simulink model "env_extQ16"  (R2022b)
settings: Solver=VariableStepAuto  StartTime=0.0  StopTime=30  RelTol=1e-3
values from neighbouring files (symbols this model uses):
  B = 8    [variables.m]    (also in variables16.m)
  cordic_delay = 20    [variables.m]    (also in variables16.m)
  e_val = 1/l2    [variables.m]    (also in variables16.m)
  exp_fract_len_homo = 26    [variables.m]    (also in variables16.m = 10)
  exp_word_len_homo = 32    [variables.m]    (also in variables16.m = 16)
  explarge_delay = 3    [variables.m]    (also in variables16.m)
  fft_len_hilb = 2048    [variables.m]    (also in variables16.m)
  fft_length = 4096    [variables.m]    (also in variables16.m)
  frac_bit_l2 = 30    [variables.m]    (also in variables16.m = 14)
  frac_bit_l3 = 29    [variables.m]    (also in variables16.m = 13)
  frac_bit_l4 = 28    [variables.m]    (also in variables16.m = 12)
  grp_delay_hilb = 11    [variables.m]    (also in variables16.m)
  grp_delay_homo = 13    [variables.m]    (also in variables16.m)
  grp_delay_psd = 19    [variables.m]    (also in variables16.m)
  grp_delay_swt = 12    [variables.m]    (also in variables16.m)
  l2 = log(2)    [variables.m]    (also in variables16.m)
  l2e = 1/log2(exp(1))    [variables.m]    (also in variables16.m)
  log2_table = log2((2^(B-1) : 2^(B)) / 2^(B - 1))    [variables.m]    (also in variables16.m)
  log_fract_len_homo = 31    [variables.m]    (also in variables16.m = 15)
  log_latency = 21    [variables.m]    (also in variables16.m)
  log_word_len = 48    [variables.m]    (also in variables16.m = 24)
  log_word_len_homo = 32    [variables.m]    (also in variables16.m = 16)
  NLZLUT = B-ceil(log2((1:2^B)))    [variables.m]    (also in variables16.m)
  scale = 1.0 / (fs * sum(window_val.*window_val))    [variables.m]    (also in variables16.m)
  win_dim = 64    [variables.m]    (also in variables16.m)
  window_dim = 100    [variables.m]    (also in variables16.m)
undefined symbols (not defined in the file or in its folder): C, c, fl_high_index, fl_low_index, HiD, hilbert_fifo_full, LoD, psd_fifo_full, SFVC784, swt_fifo_full, XCK26, xlfda_numerator
libraries: hdlBasic x626, hdlDSPIP x12, hdlUtilities x2, dspsnks4 x1, dspvision x1, vmcUtilities x1
(part 4 of 7)

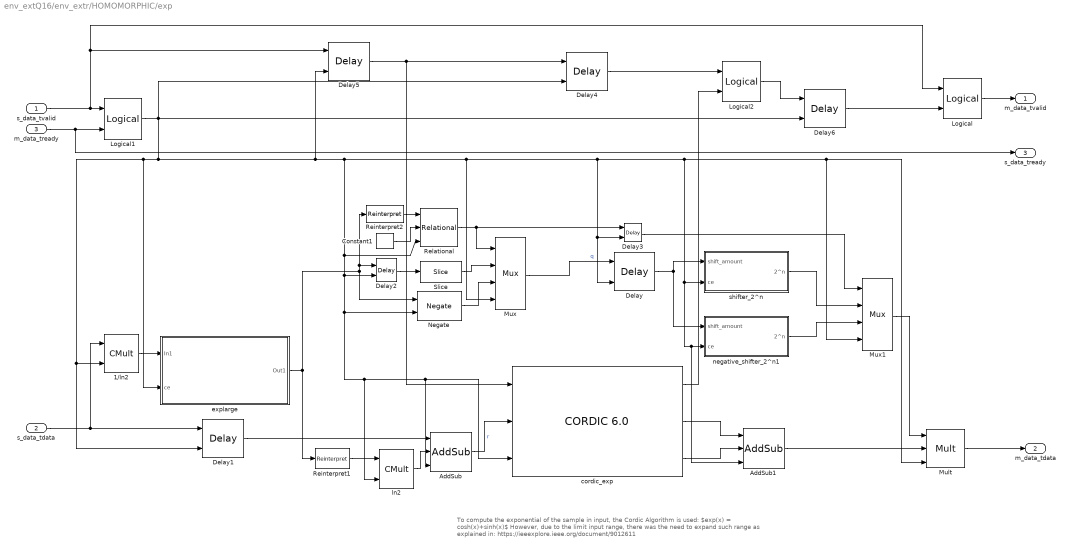
== system env_extQ16/env_extr/HOMOMORPHIC/exp ==
  note: To compute the exponential of the sample in input, the Cordic Algorithm is used: $exp(x) = cosh(x)+sinh(x)$
      |
      | However, due to the limit input range, there was the need to expand such range as explained in:
      | https://ieeexplore.ieee.org/document/9012611
  s_data_tvalid : Inport
  s_data_tdata : Inport  Port=2
  m_data_tready : Inport  Port=3
  1/ln2 : hdlBasic/CMult  const=e_val  gui_display_data_type=Fixed-point  const_n_bits=32  const_bin_pt=30  float_type=Single  exp_bits=8  fraction_bits=24  en=on  latency=1  precision=User Defined  arith_type="Signed  (2's comp)"  n_bits=exp_word_len_homo  bin_pt=exp_fract_len_homo  quantization=Truncate  overflow=Saturate  use_behavioral_HDL=off  mem_type=Distributed RAM  pipeline=off  XmcBlockStatus=1  maskContainerNames=tabcontainer1  block_type=cmult  block_config=sysgen:CMult_config
      settings: infoedit=[]
  AddSub : hdlBasic/AddSub  mode=Subtraction  use_carryin=off  use_carryout=off  en=on  latency=1  precision=User Defined  arith_type="Signed  (2's comp)"  n_bits=cordic_input_width  bin_pt=cordic_bin_point  quantization="Round  (unbiased: +/- Inf)"  overflow=Wrap  use_behavioral_HDL=off  hw_selection=Fabric  pipelined=off  XmcBlockStatus=1  maskContainerNames=tabcontainer1  block_type=addsub  block_config=sysgen:Addsub_config
  AddSub1 : hdlBasic/AddSub  mode=Addition  use_carryin=off  use_carryout=off  en=on  latency=1  precision=Full  arith_type=Unsigned  n_bits=16  bin_pt=14  quantization=Truncate  overflow=Wrap  use_behavioral_HDL=off  hw_selection=Fabric  pipelined=off  XmcBlockStatus=1  maskContainerNames=tabcontainer1  block_type=addsub  block_config=sysgen:Addsub_config
  Constant1 : hdlBasic/Constant  const=0  gui_display_data_type=Fixed-point  arith_type=Signed (2's comp)  n_bits=5  bin_pt=0  preci_type=Single  exp_width=8  frac_width=24  explicit_period=off  period=1  XmcBlockStatus=1  maskContainerNames=tabcontainer1  block_type=constant  block_config=sysgen:Constant_config
  Delay : hdlBasic/Delay  rst=off  en=on  latency=cordic_delay-2  reg_retiming=off  XmcBlockStatus=1  maskContainerNames=group1  block_type=delay  block_config=sysgen:Delay_config
  Delay1 : hdlBasic/Delay  rst=off  en=on  latency=explarge_delay+1+1  reg_retiming=off  XmcBlockStatus=1  maskContainerNames=group1  block_type=delay  block_config=sysgen:Delay_config
  Delay2 : hdlBasic/Delay  rst=off  en=on  latency=1  reg_retiming=off  XmcBlockStatus=1  maskContainerNames=group1  block_type=delay  block_config=sysgen:Delay_config
  Delay3 : hdlBasic/Delay  rst=off  en=on  latency=cordic_delay+1  reg_retiming=off  XmcBlockStatus=1  maskContainerNames=group1  block_type=delay  block_config=sysgen:Delay_config
  Delay4 : hdlBasic/Delay  rst=off  en=on  latency=cordic_delay  reg_retiming=off  XmcBlockStatus=1  maskContainerNames=group1  block_type=delay  block_config=sysgen:Delay_config
  Delay5 : hdlBasic/Delay  rst=off  en=on  latency=6  reg_retiming=off  XmcBlockStatus=1  maskContainerNames=group1  block_type=delay  block_config=sysgen:Delay_config
  Delay6 : hdlBasic/Delay  rst=off  en=on  latency=4  reg_retiming=off  XmcBlockStatus=1  maskContainerNames=group1  block_type=delay  block_config=sysgen:Delay_config
  Logical : hdlBasic/Logical  logical_function=AND  inputs=2  en=off  latency=0  precision=Full  arith_type=Unsigned  n_bits=16  bin_pt=0  align_bp=on  overflow=[]  quantization=[]  XmcBlockStatus=1  maskContainerNames=tabcontainer1  block_type=logical  block_config=sysgen:Logical_config
  Logical1 : hdlBasic/Logical  logical_function=AND  inputs=2  en=off  latency=0  precision=Full  arith_type=Unsigned  n_bits=16  bin_pt=0  align_bp=on  overflow=[]  quantization=[]  XmcBlockStatus=1  maskContainerNames=tabcontainer1  block_type=logical  block_config=sysgen:Logical_config
  Logical2 : hdlBasic/Logical  logical_function=AND  inputs=2  en=off  latency=0  precision=Full  arith_type=Unsigned  n_bits=16  bin_pt=0  align_bp=on  overflow=[]  quantization=[]  XmcBlockStatus=1  maskContainerNames=tabcontainer1  block_type=logical  block_config=sysgen:Logical_config
  Mult : hdlBasic/Mult  precision=User Defined  arith_type="Signed  (2's comp)"  n_bits=32  bin_pt=31  quantization="Round  (unbiased: +/- Inf)"  overflow=Saturate  en=on  latency=3  use_behavioral_HDL=off  opt=Speed  use_embedded=on  optimum_pipeline=off  pipeline=on  use_rpm=on  placement_style=Triangular  XmcBlockStatus=1  maskContainerNames=group1  block_type=mult  block_config=sysgen:Mult_config  block_width=598  block_height=876
  Mux : hdlBasic/Mux  inputs=2  en=on  latency=1  precision=Full  arith_type=Unsigned  n_bits=16  bin_pt=14  quantization=Truncate  overflow=Wrap  XmcBlockStatus=1  maskContainerNames=tabcontainer1  block_type=mux  block_config=sysgen:Mux_config
  Mux1 : hdlBasic/Mux  inputs=2  en=on  latency=1  precision=Full  arith_type=Unsigned  n_bits=16  bin_pt=14  quantization=Truncate  overflow=Wrap  XmcBlockStatus=1  maskContainerNames=tabcontainer1  block_type=mux  block_config=sysgen:Mux_config
  Negate : hdlBasic/Negate  precision=User Defined  arith_type=Unsigned  n_bits=5  bin_pt=0  quantization=Truncate  overflow=Wrap  en=on  latency=1  XmcBlockStatus=1  maskContainerNames=tabcontainer1  block_type=negate  block_config=sysgen:Negate_config
  Reinterpret1 : hdlBasic/Reinterpret  force_arith_type=on  arith_type="Signed  (2's comp)"  force_bin_pt=on  bin_pt=0  XmcBlockStatus=1  maskContainerNames=group1  block_type=reinterpret  block_config=sysgen:Reinterpret_config
  Reinterpret2 : hdlBasic/Reinterpret  force_arith_type=on  arith_type="Signed  (2's comp)"  force_bin_pt=on  bin_pt=0  XmcBlockStatus=1  maskContainerNames=group1  block_type=reinterpret  block_config=sysgen:Reinterpret_config
  Relational : hdlBasic/Relational  mode=a<=b  op_type=Bool  en=on  latency=1  XmcBlockStatus=1  maskContainerNames=tabcontainer1  block_type=relational  block_config=sysgen:Relational_config
  Slice : hdlBasic/Slice  nbits=5  boolean_output=off  mode=Upper Bit Location + Width  bit1=-1  base1=MSB of Input  bit0=0  base0=LSB of Input  XmcBlockStatus=1  maskContainerNames=group1  block_type=slice  block_config=sysgen:Slice_config
  cordic_exp : hdlDSPIP/CORDIC 6.0   functional_selection=Sinh_and_Cosh  architectural_configuration=Parallel  pipelining_mode=Maximum  data_format=SignedFraction  phase_format=Radians  input_width=cordic_input_width  output_width=cordic_output_width  round_mode=Nearest_Even  iterations=cordic_iterations  precision=0  compensation_scaling=No_Scale_Compensation  coarse_rotation=off  aclken=on  aresetn=off  out_tready=off  cartesian_has_tuser=off  cartesian_has_tlast=off  cartesian_tuser_width=1  phase_has_tuser=off  phase_has_tlast=off  phase_tuser_width=1  out_tlast_behv=Null  flow_control=NonBlocking  optimize_goal=Resources  trim_axipin_name=off  simulation_type=hybrid_sim  simulation_model=sysgen:cordic_v6_0  data_path_portlist={'s_axis_cartesian_tdata_imag', 's_axis_cartesian_tdata_real', 's_axis_phase_tdata_phase', 'm_axis_dout_tdata_imag', 'm_axis_dout_tdata_real', 'm_axis_dout_tdata_phase','m_axis_dout_tdata'}  ip_name=CORDIC  ip_version=6.0  dsptool_ready=true  ipcore_usecache=true  ipcore_useipmodelcache=true  wrapper_available=true  port_translation_map={ 'aclken' => 'en', 'aresetn' => 'rst' }  XmcBlockStatus=1  maskContainerNames=group15  block_type=cordic_v6_0  block_config=sysgen:rodinimport_config  block_width=800
  explarge : Subsystem
  ln2 : hdlBasic/CMult  const=l2  gui_display_data_type=Fixed-point  const_n_bits=32  const_bin_pt=31  float_type=Single  exp_bits=8  fraction_bits=24  en=on  latency=1  precision=Full  arith_type="Signed  (2's comp)"  n_bits=33  bin_pt=30  quantization="Round  (unbiased: +/- Inf)"  overflow=Wrap  use_behavioral_HDL=off  mem_type=Distributed RAM  pipeline=off  XmcBlockStatus=1  maskContainerNames=tabcontainer1  block_type=cmult  block_config=sysgen:CMult_config
      settings: infoedit=[]
  negative_shifter_2^n1 : Subsystem
  shifter_2^n : Subsystem
  m_data_tvalid : Outport
  m_data_tdata : Outport  Port=2
  s_data_tready : Outport  Port=3
  wires:
  Slice/1 -> Mux/2
  Reinterpret1/1 -> ln2/1
  s_data_tdata/1 -> 1/ln2/1, Delay1/1
  Delay/1 -> negative_shifter_2^n1/1(shift_amount), shifter_2^n/1(shift_amount)
  Delay2/1 -> Slice/1
  cordic_exp/3 -> AddSub1/2
  Constant1/1 -> Relational/2
  AddSub/1 -> cordic_exp/2  "r"
  explarge/1(Out1) -> Reinterpret1/1, Delay2/1, Reinterpret2/1, Negate/1
  Delay3/1 -> Mux1/1
  Mux1/1 -> Mult/1
  Relational/1 -> Mux/1, Delay3/1
  cordic_exp/2 -> AddSub1/1
  Negate/1 -> Mux/3
  negative_shifter_2^n1/1(2^n) -> Mux1/3
  shifter_2^n/1(2^n) -> Mux1/2
  1/ln2/1 -> explarge/1(In1)
  Mux/1 -> Delay/1  "q"
  Reinterpret2/1 -> Relational/1
  Mult/1 -> m_data_tdata/1
  AddSub1/1 -> Mult/2
  cordic_exp/1 -> Logical2/2
  m_data_tready/1 -> s_data_tready/1, Logical1/2
  s_data_tvalid/1 -> Logical/1, Delay5/1, Logical1/1
  Logical/1 -> m_data_tvalid/1
  Logical1/1 -> Delay4/2, Delay6/2, Delay1/2, 1/ln2/2, explarge/2(ce), Mux/4, Delay/2, Delay3/2, Mux1/4, Mult/3, shifter_2^n/2(ce), negative_shifter_2^n1/2(ce), AddSub1/3, ln2/2, cordic_exp/3, AddSub/3, Negate/2, Delay2/2, Relational/3, Delay5/2
  Delay4/1 -> Logical2/1
  Logical2/1 -> Delay6/1
  Delay6/1 -> Logical/2
  Delay1/1 -> AddSub/1
  ln2/1 -> AddSub/2
  Delay5/1 -> Delay4/1, cordic_exp/1

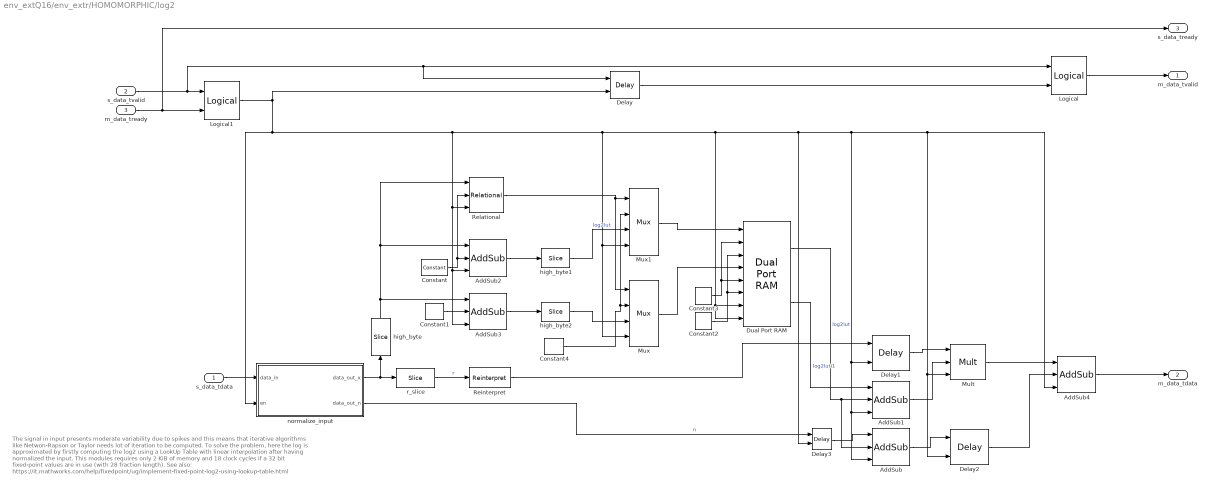
== system env_extQ16/env_extr/HOMOMORPHIC/log2 ==
  note: The signal in input presents moderate variability due to spikes and this means that iterative algorithms like Netwon-Rapson or Taylor needs lot of iteration to be computed.
      |
      | To solve the problem, here the log is approximated by firstly computing the log2 using a LookUp Table with linear interpolation after having normalized the input.
      | This modules requires only 2 KiB of memory and 18 clock cycles if a 32 bit fixed-point values are in use (with 28 fraction length).
      |
      | See also: https://it.mathworks.com/help/fixedpoint/ug/implement-fixed-point-log2-using-lookup-table.html
  s_data_tdata : Inport
  s_data_tvalid : Inport  Port=2
  m_data_tready : Inport  Port=3
  AddSub : hdlBasic/AddSub  mode=Addition  use_carryin=off  use_carryout=off  en=on  latency=1  precision=User Defined  arith_type="Signed  (2's comp)"  n_bits=32  bin_pt=25  quantization="Round  (unbiased: +/- Inf)"  overflow=Wrap  use_behavioral_HDL=off  hw_selection=Fabric  pipelined=off  XmcBlockStatus=1  maskContainerNames=tabcontainer1  block_type=addsub  block_config=sysgen:Addsub_config
  AddSub1 : hdlBasic/AddSub  mode=Subtraction  use_carryin=off  use_carryout=off  en=on  latency=1  precision=User Defined  arith_type=Unsigned  n_bits=32  bin_pt=31  quantization="Round  (unbiased: +/- Inf)"  overflow=Wrap  use_behavioral_HDL=off  hw_selection=Fabric  pipelined=off  XmcBlockStatus=1  maskContainerNames=tabcontainer1  block_type=addsub  block_config=sysgen:Addsub_config
  AddSub2 : hdlBasic/AddSub  mode=Subtraction  use_carryin=off  use_carryout=off  en=on  latency=1  precision=Full  arith_type=Unsigned  n_bits=8  bin_pt=0  quantization=Truncate  overflow=Wrap  use_behavioral_HDL=off  hw_selection=Fabric  pipelined=off  XmcBlockStatus=1  maskContainerNames=tabcontainer1  block_type=addsub  block_config=sysgen:Addsub_config
  AddSub3 : hdlBasic/AddSub  mode=Subtraction  use_carryin=off  use_carryout=off  en=on  latency=1  precision=Full  arith_type=Unsigned  n_bits=7  bin_pt=0  quantization=Truncate  overflow=Wrap  use_behavioral_HDL=off  hw_selection=Fabric  pipelined=off  XmcBlockStatus=1  maskContainerNames=tabcontainer1  block_type=addsub  block_config=sysgen:Addsub_config
  AddSub4 : hdlBasic/AddSub  mode=Addition  use_carryin=off  use_carryout=off  en=on  latency=1  precision=User Defined  arith_type="Signed  (2's comp)"  n_bits=32  bin_pt=25  quantization="Round  (unbiased: +/- Inf)"  overflow=Wrap  use_behavioral_HDL=off  hw_selection=Fabric  pipelined=off  XmcBlockStatus=1  maskContainerNames=tabcontainer1  block_type=addsub  block_config=sysgen:Addsub_config
  Constant : hdlBasic/Constant  const=2^(B-1)  gui_display_data_type=Fixed-point  arith_type=Unsigned  n_bits=ceil(log2(2^(B-1)+1))  bin_pt=0  preci_type=Single  exp_width=8  frac_width=24  explicit_period=off  period=1  XmcBlockStatus=1  maskContainerNames=tabcontainer1  block_type=constant  block_config=sysgen:Constant_config
  Constant1 : hdlBasic/Constant  const=127  gui_display_data_type=Fixed-point  arith_type=Unsigned  n_bits=ceil(log2(2^(B-1)+1))  bin_pt=0  preci_type=Single  exp_width=8  frac_width=24  explicit_period=off  period=1  XmcBlockStatus=1  maskContainerNames=tabcontainer1  block_type=constant  block_config=sysgen:Constant_config
  Constant2 : hdlBasic/Constant  const=0  gui_display_data_type=Boolean  arith_type=Boolean  n_bits=16  bin_pt=14  preci_type=Single  exp_width=8  frac_width=24  explicit_period=off  period=1  XmcBlockStatus=1  maskContainerNames=tabcontainer1  block_type=constant  block_config=sysgen:Constant_config
  Constant3 : hdlBasic/Constant  const=0  gui_display_data_type=Fixed-point  arith_type=Signed (2's comp)  n_bits=32  bin_pt=31  preci_type=Single  exp_width=8  frac_width=24  explicit_period=off  period=1  XmcBlockStatus=1  maskContainerNames=tabcontainer1  block_type=constant  block_config=sysgen:Constant_config
  Constant4 : hdlBasic/Constant  const=0  gui_display_data_type=Fixed-point  arith_type=Unsigned  n_bits=1  bin_pt=0  preci_type=Single  exp_width=8  frac_width=24  explicit_period=off  period=1  XmcBlockStatus=1  maskContainerNames=tabcontainer1  block_type=constant  block_config=sysgen:Constant_config
  Delay : hdlBasic/Delay  rst=off  en=on  latency=16  reg_retiming=off  XmcBlockStatus=1  maskContainerNames=group1  block_type=delay  block_config=sysgen:Delay_config
  Delay1 : hdlBasic/Delay  rst=off  en=on  latency=4  reg_retiming=off  XmcBlockStatus=1  maskContainerNames=group1  block_type=delay  block_config=sysgen:Delay_config
  Delay2 : hdlBasic/Delay  rst=off  en=on  latency=3  reg_retiming=off  XmcBlockStatus=1  maskContainerNames=group1  block_type=delay  block_config=sysgen:Delay_config
  Delay3 : hdlBasic/Delay  rst=off  en=on  latency=3  reg_retiming=off  XmcBlockStatus=1  maskContainerNames=group1  block_type=delay  block_config=sysgen:Delay_config
  Dual Port RAM : hdlBasic/Dual Port RAM  depth=length(log2_table)  initVector=log2_table  distributed_mem=Block RAM  init_a=0  init_b=0  rst_a=off  rst_b=off  en_a=on  en_b=on  latency=1  write_mode_A=Read After Write  write_mode_B=Read After Write  explicit_period=[]  period=[]  simulation_type=fast_sim  XmcBlockStatus=1  maskContainerNames=tabcontainer1  block_type=dpram  block_config=sysgen:Dpram_config  optimize=Area
      settings: infoedit=[]
  Logical : hdlBasic/Logical  logical_function=AND  inputs=2  en=off  latency=0  precision=Full  arith_type=Unsigned  n_bits=16  bin_pt=0  align_bp=on  overflow=[]  quantization=[]  XmcBlockStatus=1  maskContainerNames=tabcontainer1  block_type=logical  block_config=sysgen:Logical_config
  Logical1 : hdlBasic/Logical  logical_function=AND  inputs=2  en=off  latency=0  precision=Full  arith_type=Unsigned  n_bits=16  bin_pt=0  align_bp=on  overflow=[]  quantization=[]  XmcBlockStatus=1  maskContainerNames=tabcontainer1  block_type=logical  block_config=sysgen:Logical_config
  Mult : hdlBasic/Mult  precision=User Defined  arith_type="Signed  (2's comp)"  n_bits=32  bin_pt=26  quantization="Round  (unbiased: +/- Inf)"  overflow=Wrap  en=on  latency=3  use_behavioral_HDL=off  opt=Speed  use_embedded=on  optimum_pipeline=off  pipeline=on  use_rpm=on  placement_style=Triangular  XmcBlockStatus=1  maskContainerNames=group1  block_type=mult  block_config=sysgen:Mult_config  block_width=598  block_height=876
  Mux : hdlBasic/Mux  inputs=2  en=on  latency=1  precision=Full  arith_type=Unsigned  n_bits=16  bin_pt=14  quantization=Truncate  overflow=Wrap  XmcBlockStatus=1  maskContainerNames=tabcontainer1  block_type=mux  block_config=sysgen:Mux_config
  Mux1 : hdlBasic/Mux  inputs=2  en=on  latency=1  precision=Full  arith_type=Unsigned  n_bits=16  bin_pt=14  quantization=Truncate  overflow=Wrap  XmcBlockStatus=1  maskContainerNames=tabcontainer1  block_type=mux  block_config=sysgen:Mux_config
  Reinterpret : hdlBasic/Reinterpret  force_arith_type=on  arith_type=Unsigned  force_bin_pt=on  bin_pt=log_word_len_homo-B  XmcBlockStatus=1  maskContainerNames=group1  block_type=reinterpret  block_config=sysgen:Reinterpret_config
  Relational : hdlBasic/Relational  mode=a>=b  op_type=Bool  en=on  latency=1  XmcBlockStatus=1  maskContainerNames=tabcontainer1  block_type=relational  block_config=sysgen:Relational_config
  high_byte : hdlBasic/Slice  nbits=B  boolean_output=off  mode=Upper Bit Location + Width  bit1=0  base1=MSB of Input  bit0=0  base0=LSB of Input  XmcBlockStatus=1  maskContainerNames=group1  block_type=slice  block_config=sysgen:Slice_config
  high_byte1 : hdlBasic/Slice  nbits=B  boolean_output=off  mode=Upper Bit Location + Width  bit1=-1  base1=MSB of Input  bit0=0  base0=LSB of Input  XmcBlockStatus=1  maskContainerNames=group1  block_type=slice  block_config=sysgen:Slice_config
  high_byte2 : hdlBasic/Slice  nbits=B  boolean_output=off  mode=Upper Bit Location + Width  bit1=-1  base1=MSB of Input  bit0=0  base0=LSB of Input  XmcBlockStatus=1  maskContainerNames=group1  block_type=slice  block_config=sysgen:Slice_config
  normalize_input : Subsystem
  r_slice : hdlBasic/Slice  nbits=log_word_len_homo-B  boolean_output=off  mode=Upper Bit Location + Width  bit1=-B  base1=MSB of Input  bit0=0  base0=LSB of Input  XmcBlockStatus=1  maskContainerNames=group1  block_type=slice  block_config=sysgen:Slice_config
  m_data_tvalid : Outport
  m_data_tdata : Outport  Port=2
  s_data_tready : Outport  Port=3
  wires:
  normalize_input/1(data_out_x) -> r_slice/1, high_byte/1
  Dual Port RAM/1 -> AddSub/2, AddSub1/2  "log2lut"
  r_slice/1 -> Reinterpret/1  "r"
  s_data_tdata/1 -> normalize_input/1(data_in)
  Constant1/1 -> AddSub3/2
  AddSub2/1 -> high_byte1/1
  AddSub1/1 -> Mult/2
  AddSub3/1 -> high_byte2/1
  Dual Port RAM/2 -> AddSub1/1  "log2luti1"
  Constant/1 -> Relational/2, AddSub2/2
  AddSub/1 -> Delay2/1
  normalize_input/2(data_out_n) -> Delay3/1  "n"
  Delay1/1 -> Mult/1
  Mult/1 -> AddSub4/1
  Delay2/1 -> AddSub4/2
  AddSub4/1 -> m_data_tdata/1
  high_byte/1 -> AddSub3/1, Relational/1, AddSub2/1
  Reinterpret/1 -> Delay1/1
  Delay3/1 -> AddSub/1
  Constant2/1 -> Dual Port RAM/3, Dual Port RAM/6
  Constant3/1 -> Dual Port RAM/2, Dual Port RAM/5
  high_byte1/1 -> Mux1/3  "log2lut"
  high_byte2/1 -> Mux/3
  Mux1/1 -> Dual Port RAM/1
  Mux/1 -> Dual Port RAM/4
  Relational/1 -> Mux/1, Mux1/1
  Constant4/1 -> Mux1/2, Mux/2
  s_data_tvalid/1 -> Logical1/1, Delay/1, Logical/1
  m_data_tready/1 -> s_data_tready/1, Logical1/2
  Logical/1 -> m_data_tvalid/1
  Logical1/1 -> AddSub3/3, AddSub2/3, Relational/3, Mux/4, Mux1/4, Dual Port RAM/8, Dual Port RAM/7, Delay3/2, AddSub1/3, AddSub/3, Delay1/2, AddSub4/3, Delay2/2, Mult/3, normalize_input/2(en), Delay/2
  Delay/1 -> Logical/2

== system env_extQ16/env_extr/SWT/Level-2 ==
  data_s_tdata : Inport
  s_data_tvalid : Inport  Port=2
  m_data_tready : Inport  Port=3
  AddSub2 : hdlBasic/AddSub  mode=Addition  use_carryin=off  use_carryout=off  en=on  latency=1  precision=User Defined  arith_type="Signed  (2's comp)"  n_bits=bit_width_l2  bin_pt=frac_bit_l2-1  quantization="Round  (unbiased: +/- Inf)"  overflow=Saturate  use_behavioral_HDL=off  hw_selection=Fabric  pipelined=off  XmcBlockStatus=1  maskContainerNames=tabcontainer1  block_type=addsub  block_config=sysgen:Addsub_config
  AddSub4 : hdlBasic/AddSub  mode=Addition  use_carryin=off  use_carryout=off  en=on  latency=1  precision=User Defined  arith_type="Signed  (2's comp)"  n_bits=bit_width_l2  bin_pt=frac_bit_l2  quantization="Round  (unbiased: +/- Inf)"  overflow=Wrap  use_behavioral_HDL=off  hw_selection=Fabric  pipelined=off  XmcBlockStatus=1  maskContainerNames=tabcontainer1  block_type=addsub  block_config=sysgen:Addsub_config
  AddSub6 : hdlBasic/AddSub  mode=Addition  use_carryin=off  use_carryout=off  en=on  latency=1  precision=User Defined  arith_type="Signed  (2's comp)"  n_bits=bit_width_l2  bin_pt=frac_bit_l2  quantization="Round  (unbiased: +/- Inf)"  overflow=Wrap  use_behavioral_HDL=off  hw_selection=Fabric  pipelined=off  XmcBlockStatus=1  maskContainerNames=tabcontainer1  block_type=addsub  block_config=sysgen:Addsub_config
  CMult : hdlBasic/CMult  const=LoD(1)  gui_display_data_type=Fixed-point  const_n_bits=const_bin_width  const_bin_pt=const_frac_width  float_type=Single  exp_bits=8  fraction_bits=24  en=on  latency=1  precision=User Defined  arith_type="Signed  (2's comp)"  n_bits=bit_width_l2  bin_pt=frac_bit_l2  quantization="Round  (unbiased: +/- Inf)"  overflow=Wrap  use_behavioral_HDL=off  mem_type=Distributed RAM  pipeline=off  XmcBlockStatus=1  maskContainerNames=tabcontainer1  block_type=cmult  block_config=sysgen:CMult_config
      settings: infoedit=[]
  CMult1 : hdlBasic/CMult  const=0  gui_display_data_type=Fixed-point  const_n_bits=const_bin_width  const_bin_pt=const_frac_width  float_type=Single  exp_bits=8  fraction_bits=24  en=on  latency=1  precision=User Defined  arith_type="Signed  (2's comp)"  n_bits=bit_width_l2  bin_pt=frac_bit_l2  quantization=Truncate  overflow=Wrap  use_behavioral_HDL=off  mem_type=Distributed RAM  pipeline=off  XmcBlockStatus=1  maskContainerNames=tabcontainer1  block_type=cmult  block_config=sysgen:CMult_config
      settings: infoedit=[]
  CMult2 : hdlBasic/CMult  const=LoD(2)  gui_display_data_type=Fixed-point  const_n_bits=const_bin_width  const_bin_pt=const_frac_width  float_type=Single  exp_bits=8  fraction_bits=24  en=on  latency=1  precision=User Defined  arith_type="Signed  (2's comp)"  n_bits=bit_width_l2  bin_pt=frac_bit_l2  quantization="Round  (unbiased: +/- Inf)"  overflow=Wrap  use_behavioral_HDL=off  mem_type=Distributed RAM  pipeline=off  XmcBlockStatus=1  maskContainerNames=tabcontainer1  block_type=cmult  block_config=sysgen:CMult_config
      settings: infoedit=[]
  CMult3 : hdlBasic/CMult  const=0  gui_display_data_type=Fixed-point  const_n_bits=const_bin_width  const_bin_pt=const_frac_width  float_type=Single  exp_bits=8  fraction_bits=24  en=on  latency=1  precision=User Defined  arith_type="Signed  (2's comp)"  n_bits=bit_width_l2  bin_pt=frac_bit_l2  quantization=Truncate  overflow=Wrap  use_behavioral_HDL=off  mem_type=Distributed RAM  pipeline=off  XmcBlockStatus=1  maskContainerNames=tabcontainer1  block_type=cmult  block_config=sysgen:CMult_config
      settings: infoedit=[]
  Delay{1..6} (6 alike) : hdlBasic/Delay  rst=off  en=on  latency=1  reg_retiming=off  XmcBlockStatus=1  maskContainerNames=group1  block_type=delay  block_config=sysgen:Delay_config
  Logical : hdlBasic/Logical  logical_function=AND  inputs=2  en=off  latency=0  precision=Full  arith_type=Unsigned  n_bits=16  bin_pt=0  align_bp=on  overflow=[]  quantization=[]  XmcBlockStatus=1  maskContainerNames=tabcontainer1  block_type=logical  block_config=sysgen:Logical_config
  Logical1 : hdlBasic/Logical  logical_function=AND  inputs=2  en=off  latency=0  precision=Full  arith_type=Unsigned  n_bits=16  bin_pt=0  align_bp=on  overflow=[]  quantization=[]  XmcBlockStatus=1  maskContainerNames=tabcontainer1  block_type=logical  block_config=sysgen:Logical_config
  m_data_tdata : Outport
  m_data_tvalid : Outport  Port=2
  s_data_tready : Outport  Port=3
  wires:
  Delay5/1 -> CMult3/1
  Delay4/1 -> CMult2/1, Delay5/1
  Delay3/1 -> CMult1/1, Delay4/1
  data_s_tdata/1 -> CMult/1, Delay3/1
  CMult3/1 -> AddSub6/2
  CMult1/1 -> AddSub4/2
  CMult2/1 -> AddSub6/1
  AddSub6/1 -> AddSub2/2
  AddSub2/1 -> m_data_tdata/1
  AddSub4/1 -> AddSub2/1
  CMult/1 -> AddSub4/1
  Delay1/1 -> Delay2/1
  Delay2/1 -> Delay6/1
  s_data_tvalid/1 -> Logical1/2, Delay1/1, Logical/1
  m_data_tready/1 -> s_data_tready/1, Logical/2
  Logical/1 -> Delay6/2, Delay2/2, Delay1/2, CMult3/2, AddSub6/3, CMult2/2, AddSub2/3, CMult1/2, AddSub4/3, CMult/2, Delay3/2, Delay4/2, Delay5/2
  Logical1/1 -> m_data_tvalid/1
  Delay6/1 -> Logical1/1

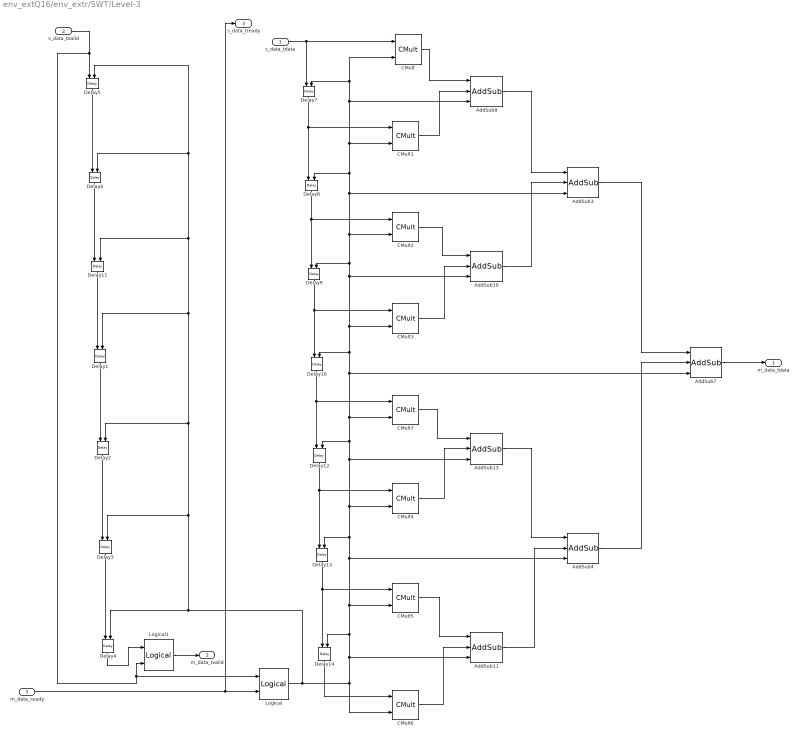
== system env_extQ16/env_extr/SWT/Level-3 ==
  s_data_tdata : Inport
  s_data_tvalid : Inport  Port=2
  m_data_ready : Inport  Port=3
  AddSub10 : hdlBasic/AddSub  mode=Addition  use_carryin=off  use_carryout=off  en=on  latency=1  precision=User Defined  arith_type="Signed  (2's comp)"  n_bits=bit_width_l3  bin_pt=frac_bit_l3  quantization=Truncate  overflow=Wrap  use_behavioral_HDL=off  hw_selection=Fabric  pipelined=off  XmcBlockStatus=1  maskContainerNames=tabcontainer1  block_type=addsub  block_config=sysgen:Addsub_config
  AddSub11 : hdlBasic/AddSub  mode=Addition  use_carryin=off  use_carryout=off  en=on  latency=1  precision=User Defined  arith_type="Signed  (2's comp)"  n_bits=bit_width_l3  bin_pt=frac_bit_l3  quantization=Truncate  overflow=Wrap  use_behavioral_HDL=off  hw_selection=Fabric  pipelined=off  XmcBlockStatus=1  maskContainerNames=tabcontainer1  block_type=addsub  block_config=sysgen:Addsub_config
  AddSub{3..4,8,13} (4 alike) : hdlBasic/AddSub  mode=Addition  use_carryin=off  use_carryout=off  en=on  latency=1  precision=User Defined  arith_type="Signed  (2's comp)"  n_bits=bit_width_l3  bin_pt=frac_bit_l3  quantization="Round  (unbiased: +/- Inf)"  overflow=Wrap  use_behavioral_HDL=off  hw_selection=Fabric  pipelined=off  XmcBlockStatus=1  maskContainerNames=tabcontainer1  block_type=addsub  block_config=sysgen:Addsub_config
  AddSub7 : hdlBasic/AddSub  mode=Addition  use_carryin=off  use_carryout=off  en=on  latency=1  precision=User Defined  arith_type="Signed  (2's comp)"  n_bits=bit_width_l3  bin_pt=frac_bit_l3-1  quantization="Round  (unbiased: +/- Inf)"  overflow=Saturate  use_behavioral_HDL=off  hw_selection=Fabric  pipelined=off  XmcBlockStatus=1  maskContainerNames=tabcontainer1  block_type=addsub  block_config=sysgen:Addsub_config
  CMult : hdlBasic/CMult  const=LoD(1)  gui_display_data_type=Fixed-point  const_n_bits=const_bin_width  const_bin_pt=const_frac_width  float_type=Single  exp_bits=8  fraction_bits=24  en=on  latency=1  precision=User Defined  arith_type="Signed  (2's comp)"  n_bits=bit_width_l3  bin_pt=frac_bit_l3  quantization="Round  (unbiased: +/- Inf)"  overflow=Wrap  use_behavioral_HDL=off  mem_type=Distributed RAM  pipeline=off  XmcBlockStatus=1  maskContainerNames=tabcontainer1  block_type=cmult  block_config=sysgen:CMult_config
      settings: infoedit=[]
  CMult{1..6} (6 alike) : hdlBasic/CMult  const=0  gui_display_data_type=Fixed-point  const_n_bits=const_bin_width  const_bin_pt=const_frac_width  float_type=Single  exp_bits=8  fraction_bits=24  en=on  latency=1  precision=User Defined  arith_type="Signed  (2's comp)"  n_bits=bit_width_l3  bin_pt=frac_bit_l3  quantization=Truncate  overflow=Wrap  use_behavioral_HDL=off  mem_type=Distributed RAM  pipeline=off  XmcBlockStatus=1  maskContainerNames=tabcontainer1  block_type=cmult  block_config=sysgen:CMult_config
      settings: infoedit=[]
  CMult7 : hdlBasic/CMult  const=LoD(2)  gui_display_data_type=Fixed-point  const_n_bits=const_bin_width  const_bin_pt=const_frac_width  float_type=Single  exp_bits=8  fraction_bits=24  en=on  latency=1  precision=User Defined  arith_type="Signed  (2's comp)"  n_bits=bit_width_l3  bin_pt=frac_bit_l3  quantization="Round  (unbiased: +/- Inf)"  overflow=Wrap  use_behavioral_HDL=off  mem_type=Distributed RAM  pipeline=off  XmcBlockStatus=1  maskContainerNames=tabcontainer1  block_type=cmult  block_config=sysgen:CMult_config
      settings: infoedit=[]
  Delay{1..14} (14 alike) : hdlBasic/Delay  rst=off  en=on  latency=1  reg_retiming=off  XmcBlockStatus=1  maskContainerNames=group1  block_type=delay  block_config=sysgen:Delay_config
  Logical : hdlBasic/Logical  logical_function=AND  inputs=2  en=off  latency=0  precision=Full  arith_type=Unsigned  n_bits=16  bin_pt=0  align_bp=on  overflow=[]  quantization=[]  XmcBlockStatus=1  maskContainerNames=tabcontainer1  block_type=logical  block_config=sysgen:Logical_config
  Logical1 : hdlBasic/Logical  logical_function=AND  inputs=2  en=off  latency=0  precision=Full  arith_type=Unsigned  n_bits=16  bin_pt=0  align_bp=on  overflow=[]  quantization=[]  XmcBlockStatus=1  maskContainerNames=tabcontainer1  block_type=logical  block_config=sysgen:Logical_config
  m_data_tdata : Outport
  m_data_tvalid : Outport  Port=2
  s_data_tready : Outport  Port=3
  wires:
  Delay9/1 -> Delay10/1, CMult3/1
  CMult4/1 -> AddSub13/2
  Delay10/1 -> Delay12/1, CMult7/1
  Delay13/1 -> Delay14/1, CMult5/1
  Delay12/1 -> Delay13/1, CMult4/1
  Delay8/1 -> Delay9/1, CMult2/1
  CMult6/1 -> AddSub11/2
  Delay7/1 -> Delay8/1, CMult1/1
  CMult1/1 -> AddSub8/2
  s_data_tdata/1 -> Delay7/1, CMult/1
  CMult3/1 -> AddSub10/2
  AddSub10/1 -> AddSub3/2
  AddSub11/1 -> AddSub4/2
  AddSub7/1 -> m_data_tdata/1
  CMult2/1 -> AddSub10/1
  CMult7/1 -> AddSub13/1
  CMult5/1 -> AddSub11/1
  AddSub8/1 -> AddSub3/1
  AddSub13/1 -> AddSub4/1
  AddSub3/1 -> AddSub7/1
  AddSub4/1 -> AddSub7/2
  CMult/1 -> AddSub8/1
  Delay14/1 -> CMult6/1
  Delay1/1 -> Delay2/1
  Delay11/1 -> Delay1/1
  Delay6/1 -> Delay11/1
  Delay2/1 -> Delay3/1
  s_data_tvalid/1 -> Logical1/2, Logical/1, Delay5/1
  Delay3/1 -> Delay4/1
  Delay5/1 -> Delay6/1
  m_data_ready/1 -> Logical/2, s_data_tready/1
  Logical/1 -> Delay4/2, Delay3/2, Delay2/2, Delay1/2, Delay11/2, Delay5/2, Delay6/2, CMult6/2, AddSub11/3, Delay14/2, CMult5/2, AddSub4/3, Delay13/2, AddSub13/3, Delay12/2, CMult7/2, AddSub7/3, Delay10/2, CMult3/2, AddSub10/3, Delay9/2, AddSub3/3, Delay8/2, CMult1/2, AddSub8/3, Delay7/2, CMult/2, CMult2/2, CMult4/2
  Delay4/1 -> Logical1/1
  Logical1/1 -> m_data_tvalid/1

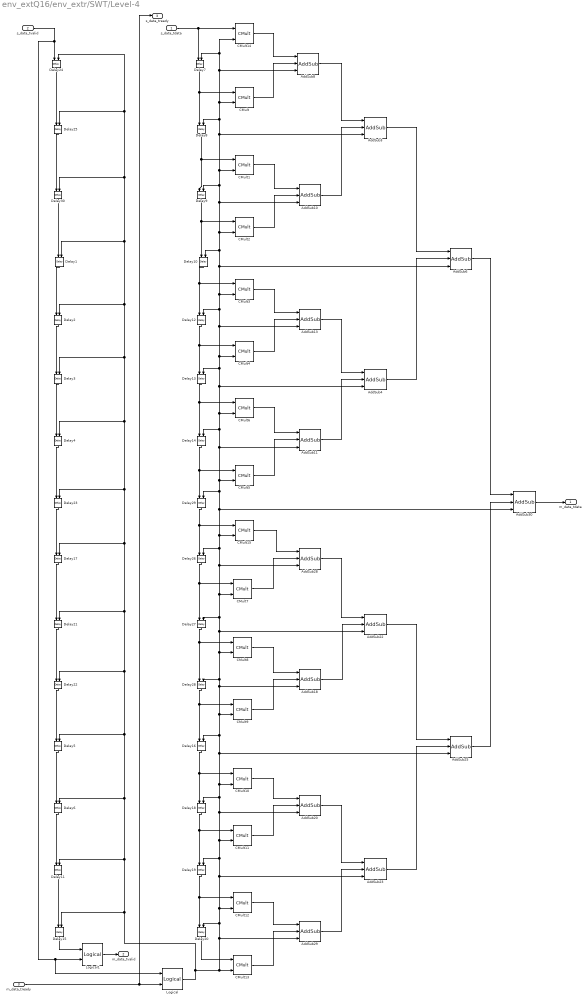
== system env_extQ16/env_extr/SWT/Level-4 ==
  s_data_tdata : Inport
  s_data_tvalid : Inport  Port=2
  m_data_tready : Inport  Port=3
  AddSub{4,10..11,18,20,23,29} (7 alike) : hdlBasic/AddSub  mode=Addition  use_carryin=off  use_carryout=off  en=on  latency=1  precision=User Defined  arith_type="Signed  (2's comp)"  n_bits=bit_width_l4  bin_pt=frac_bit_l4  quantization=Truncate  overflow=Wrap  use_behavioral_HDL=off  hw_selection=Fabric  pipelined=off  XmcBlockStatus=1  maskContainerNames=tabcontainer1  block_type=addsub  block_config=sysgen:Addsub_config
  AddSub13 : hdlBasic/AddSub  mode=Addition  use_carryin=off  use_carryout=off  en=on  latency=1  precision=User Defined  arith_type=Unsigned  n_bits=bit_width_l4  bin_pt=frac_bit_l4  quantization=Truncate  overflow=Wrap  use_behavioral_HDL=off  hw_selection=Fabric  pipelined=off  XmcBlockStatus=1  maskContainerNames=tabcontainer1  block_type=addsub  block_config=sysgen:Addsub_config
  AddSub{3,6,8,22,25} (5 alike) : hdlBasic/AddSub  mode=Addition  use_carryin=off  use_carryout=off  en=on  latency=1  precision=User Defined  arith_type="Signed  (2's comp)"  n_bits=bit_width_l4  bin_pt=frac_bit_l4  quantization="Round  (unbiased: +/- Inf)"  overflow=Wrap  use_behavioral_HDL=off  hw_selection=Fabric  pipelined=off  XmcBlockStatus=1  maskContainerNames=tabcontainer1  block_type=addsub  block_config=sysgen:Addsub_config
  AddSub28 : hdlBasic/AddSub  mode=Addition  use_carryin=off  use_carryout=off  en=on  latency=1  precision=User Defined  arith_type=Unsigned  n_bits=bit_width_l4  bin_pt=frac_bit_l4  quantization="Round  (unbiased: +/- Inf)"  overflow=Wrap  use_behavioral_HDL=off  hw_selection=Fabric  pipelined=off  XmcBlockStatus=1  maskContainerNames=tabcontainer1  block_type=addsub  block_config=sysgen:Addsub_config
  AddSub30 : hdlBasic/AddSub  mode=Addition  use_carryin=off  use_carryout=off  en=on  latency=1  precision=User Defined  arith_type="Signed  (2's comp)"  n_bits=bit_width_l4  bin_pt=frac_bit_l4-1  quantization="Round  (unbiased: +/- Inf)"  overflow=Saturate  use_behavioral_HDL=off  hw_selection=Fabric  pipelined=off  XmcBlockStatus=1  maskContainerNames=tabcontainer1  block_type=addsub  block_config=sysgen:Addsub_config
  CMult{,1..13} (14 alike) : hdlBasic/CMult  const=0  gui_display_data_type=Fixed-point  const_n_bits=const_bin_width  const_bin_pt=const_frac_width  float_type=Single  exp_bits=8  fraction_bits=24  en=on  latency=1  precision=User Defined  arith_type="Signed  (2's comp)"  n_bits=bit_width_l4  bin_pt=frac_bit_l4  quantization=Truncate  overflow=Wrap  use_behavioral_HDL=off  mem_type=Distributed RAM  pipeline=off  XmcBlockStatus=1  maskContainerNames=tabcontainer1  block_type=cmult  block_config=sysgen:CMult_config
      settings: infoedit=[]
  CMult14 : hdlBasic/CMult  const=HiD(1)  gui_display_data_type=Fixed-point  const_n_bits=const_bin_width  const_bin_pt=const_frac_width  float_type=Single  exp_bits=8  fraction_bits=24  en=on  latency=1  precision=User Defined  arith_type="Signed  (2's comp)"  n_bits=bit_width_l4  bin_pt=frac_bit_l4  quantization="Round  (unbiased: +/- Inf)"  overflow=Wrap  use_behavioral_HDL=off  mem_type=Distributed RAM  pipeline=off  XmcBlockStatus=1  maskContainerNames=tabcontainer1  block_type=cmult  block_config=sysgen:CMult_config
      settings: infoedit=[]
  CMult15 : hdlBasic/CMult  const=HiD(2)  gui_display_data_type=Fixed-point  const_n_bits=const_bin_width  const_bin_pt=const_frac_width  float_type=Single  exp_bits=8  fraction_bits=24  en=on  latency=1  precision=User Defined  arith_type="Signed  (2's comp)"  n_bits=bit_width_l4  bin_pt=frac_bit_l4  quantization="Round  (unbiased: +/- Inf)"  overflow=Wrap  use_behavioral_HDL=off  mem_type=Distributed RAM  pipeline=off  XmcBlockStatus=1  maskContainerNames=tabcontainer1  block_type=cmult  block_config=sysgen:CMult_config
      settings: infoedit=[]
  Delay{1..30} (30 alike) : hdlBasic/Delay  rst=off  en=on  latency=1  reg_retiming=off  XmcBlockStatus=1  maskContainerNames=group1  block_type=delay  block_config=sysgen:Delay_config
  Logical : hdlBasic/Logical  logical_function=AND  inputs=2  en=off  latency=0  precision=Full  arith_type=Unsigned  n_bits=16  bin_pt=0  align_bp=on  overflow=[]  quantization=[]  XmcBlockStatus=1  maskContainerNames=tabcontainer1  block_type=logical  block_config=sysgen:Logical_config
  Logical1 : hdlBasic/Logical  logical_function=AND  inputs=2  en=off  latency=0  precision=Full  arith_type=Unsigned  n_bits=16  bin_pt=0  align_bp=on  overflow=[]  quantization=[]  XmcBlockStatus=1  maskContainerNames=tabcontainer1  block_type=logical  block_config=sysgen:Logical_config
  m_data_tdata : Outport
  m_data_tvalid : Outport  Port=2
  s_data_tready : Outport  Port=3
  wires:
  CMult2/1 -> AddSub10/2
  Delay10/1 -> CMult3/1, Delay12/1
  CMult/1 -> AddSub8/2
  Delay8/1 -> Delay9/1, CMult1/1
  Delay12/1 -> CMult4/1, Delay13/1
  Delay7/1 -> CMult/1, Delay8/1
  AddSub10/1 -> AddSub3/2
  s_data_tdata/1 -> CMult14/1, Delay7/1
  CMult5/1 -> AddSub11/2
  Delay9/1 -> Delay10/1, CMult2/1
  CMult4/1 -> AddSub13/2
  Delay13/1 -> CMult6/1, Delay14/1
  AddSub3/1 -> AddSub6/1
  Delay14/1 -> CMult5/1, Delay29/1
  AddSub4/1 -> AddSub6/2
  AddSub11/1 -> AddSub4/2
  CMult14/1 -> AddSub8/1
  Delay20/1 -> CMult13/1
  Delay19/1 -> CMult12/1, Delay20/1
  AddSub18/1 -> AddSub22/2
  Delay18/1 -> CMult11/1, Delay19/1
  Delay28/1 -> CMult9/1, Delay16/1
  Delay26/1 -> CMult7/1, Delay27/1
  Delay27/1 -> CMult8/1, Delay28/1
  Delay16/1 -> CMult10/1, Delay18/1
  Delay29/1 -> CMult15/1, Delay26/1
  CMult13/1 -> AddSub29/2
  AddSub29/1 -> AddSub23/2
  AddSub23/1 -> AddSub25/2
  AddSub30/1 -> m_data_tdata/1
  CMult1/1 -> AddSub10/1
  CMult3/1 -> AddSub13/1
  CMult15/1 -> AddSub28/1
  CMult10/1 -> AddSub20/1
  CMult12/1 -> AddSub29/1
  AddSub8/1 -> AddSub3/1
  AddSub13/1 -> AddSub4/1
  AddSub28/1 -> AddSub22/1
  AddSub20/1 -> AddSub23/1
  AddSub22/1 -> AddSub25/1
  AddSub6/1 -> AddSub30/1
  AddSub25/1 -> AddSub30/2
  CMult6/1 -> AddSub11/1
  CMult7/1 -> AddSub28/2
  CMult8/1 -> AddSub18/1
  CMult9/1 -> AddSub18/2
  CMult11/1 -> AddSub20/2
  Delay4/1 -> Delay23/1
  Delay21/1 -> Delay22/1
  Delay24/1 -> Delay25/1
  Delay11/1 -> Delay15/1
  Delay23/1 -> Delay17/1
  Delay17/1 -> Delay21/1
  Delay3/1 -> Delay4/1
  Delay30/1 -> Delay1/1
  Delay6/1 -> Delay11/1
  s_data_tvalid/1 -> Logical/1, Logical1/2, Delay24/1
  Delay25/1 -> Delay30/1
  Delay22/1 -> Delay5/1
  Delay5/1 -> Delay6/1
  Delay2/1 -> Delay3/1
  Delay1/1 -> Delay2/1
  m_data_tready/1 -> s_data_tready/1, Logical/2
  Logical/1 -> Delay15/2, Delay11/2, Delay6/2, Delay5/2, Delay22/2, Delay21/2, Delay17/2, Delay23/2, Delay4/2, Delay3/2, Delay2/2, Delay1/2, Delay30/2, Delay25/2, Delay24/2, Delay20/2, CMult12/2, AddSub23/3, Delay19/2, CMult11/2, AddSub20/3, Delay18/2, CMult10/2, AddSub25/3, Delay16/2, CMult9/2, Delay28/2, CMult8/2, AddSub22/3, Delay27/2, CMult7/2, AddSub28/3, Delay26/2, CMult15/2, AddSub30/3, Delay29/2, CMult5/2, AddSub11/3, Delay14/2, CMult6/2, AddSub4/3, Delay13/2, CMult4/2, AddSub13/3, Delay12/2, CMult3/2, AddSub6/3, Delay10/2, CMult2/2, AddSub10/3, Delay9/2, CMult1/2, AddSub3/3, Delay8/2, CMult/2, AddSub8/3, Delay7/2, CMult14/2, AddSub18/3, AddSub29/3, CMult13/2
  Logical1/1 -> m_data_tvalid/1
  Delay15/1 -> Logical1/1

== system env_extQ16/env_extr/SWT/shannonE ==
  note: Here the Shannon Energy is computed as:
      | $S.E. = -x^{2}\times ln(x^{2})$
      |
      | To avoid numerical problems in computing the log, if a sample is zero, it is substituted with a small constant.
  s_data_tdata : Inport
  s_data_tvalid : Inport  Port=2
  m_data_tready : Inport  Port=3
  CMult : hdlBasic/CMult  const=l2e  gui_display_data_type=Fixed-point  const_n_bits=32  const_bin_pt=31  float_type=Single  exp_bits=8  fraction_bits=24  en=on  latency=1  precision=User Defined  arith_type="Signed  (2's comp)"  n_bits=32  bin_pt=25  quantization="Round  (unbiased: +/- Inf)"  overflow=Wrap  use_behavioral_HDL=off  mem_type=Distributed RAM  pipeline=off  XmcBlockStatus=1  maskContainerNames=tabcontainer1  block_type=cmult  block_config=sysgen:CMult_config
      settings: infoedit=[]
  Constant : hdlBasic/Constant  const=1e-8  gui_display_data_type=Fixed-point  arith_type=Signed (2's comp)  n_bits=32  bin_pt=27  preci_type=Single  exp_width=8  frac_width=24  explicit_period=off  period=1  XmcBlockStatus=1  maskContainerNames=tabcontainer1  block_type=constant  block_config=sysgen:Constant_config
  Constant1 : hdlBasic/Constant  const=0  gui_display_data_type=Fixed-point  arith_type=Signed (2's comp)  n_bits=32  bin_pt=27  preci_type=Single  exp_width=8  frac_width=24  explicit_period=off  period=1  XmcBlockStatus=1  maskContainerNames=tabcontainer1  block_type=constant  block_config=sysgen:Constant_config
  Delay : hdlBasic/Delay  rst=off  en=on  latency=log_latency  reg_retiming=off  XmcBlockStatus=1  maskContainerNames=group1  block_type=delay  block_config=sysgen:Delay_config
  Delay1 : hdlBasic/Delay  rst=off  en=on  latency=1  reg_retiming=off  XmcBlockStatus=1  maskContainerNames=group1  block_type=delay  block_config=sysgen:Delay_config
  Delay2 : hdlBasic/Delay  rst=off  en=on  latency=log_latency+9  reg_retiming=off  XmcBlockStatus=1  maskContainerNames=group1  block_type=delay  block_config=sysgen:Delay_config
  Logical : hdlBasic/Logical  logical_function=AND  inputs=2  en=off  latency=0  precision=Full  arith_type=Unsigned  n_bits=16  bin_pt=0  align_bp=on  overflow=[]  quantization=[]  XmcBlockStatus=1  maskContainerNames=tabcontainer1  block_type=logical  block_config=sysgen:Logical_config
  Logical1 : hdlBasic/Logical  logical_function=AND  inputs=2  en=off  latency=0  precision=Full  arith_type=Unsigned  n_bits=16  bin_pt=0  align_bp=on  overflow=[]  quantization=[]  XmcBlockStatus=1  maskContainerNames=tabcontainer1  block_type=logical  block_config=sysgen:Logical_config
  Mult : hdlBasic/Mult  precision=User Defined  arith_type="Signed  (2's comp)"  n_bits=log_word_len  bin_pt=log_fract_len  quantization="Round  (unbiased: +/- Inf)"  overflow=Wrap  en=on  latency=3  use_behavioral_HDL=off  opt=Speed  use_embedded=on  optimum_pipeline=off  pipeline=on  use_rpm=on  placement_style=Triangular  XmcBlockStatus=1  maskContainerNames=group1  block_type=mult  block_config=sysgen:Mult_config  block_width=598  block_height=876
  Mult1 : hdlBasic/Mult  precision=User Defined  arith_type="Signed  (2's comp)"  n_bits=32  bin_pt=25  quantization="Round  (unbiased: +/- Inf)"  overflow=Wrap  en=on  latency=3  use_behavioral_HDL=off  opt=Speed  use_embedded=on  optimum_pipeline=off  pipeline=on  use_rpm=on  placement_style=Triangular  XmcBlockStatus=1  maskContainerNames=group1  block_type=mult  block_config=sysgen:Mult_config  block_width=598  block_height=876
  Mux : hdlBasic/Mux  inputs=2  en=on  latency=1  precision=Full  arith_type=Unsigned  n_bits=16  bin_pt=14  quantization=Truncate  overflow=Wrap  XmcBlockStatus=1  maskContainerNames=tabcontainer1  block_type=mux  block_config=sysgen:Mux_config
  Negate : hdlBasic/Negate  precision=User Defined  arith_type="Signed  (2's comp)"  n_bits=32  bin_pt=25  quantization="Round  (unbiased: +/- Inf)"  overflow=Wrap  en=on  latency=1  XmcBlockStatus=1  maskContainerNames=tabcontainer1  block_type=negate  block_config=sysgen:Negate_config
  Relational : hdlBasic/Relational  mode=a=b  op_type=Bool  en=on  latency=1  XmcBlockStatus=1  maskContainerNames=tabcontainer1  block_type=relational  block_config=sysgen:Relational_config
  log2 : Subsystem
      settings: PortSchema="{\"entries\":[{\"content\":{\"sides\":[{\"content\":{\"connectorIds\":[\"In1\"]},\"type\":\"ConnectorPlacement.EquallySpacedRectSide\",\"uuid\":\"ac5ce324-0f5d-4cf4-b223-45bbd3e1d42e\"},{\"content\":{\"connectorIds\":[\"Out1\"],\"side\":\"RIGHT\"},\"type\":\"ConnectorPlacement.EquallySpacedRectSide\",\"uuid\":\"d904f2a9-75f2-462f-bbd3-fe78b37bc13f\"},{\"content\":{\"connectorIds\":[],\"side\":\"TOP\"},\"type\":\"ConnectorPlacement.EquallySpacedRectSide\",\"uuid\":\"3636fa92-f3c9-41db-9a8c-e9c0f4c4d94c\"},{\"content\":{\"connectorIds\":[\"In2\"],\"side\":\"BOTTOM\"},\"type\":\"ConnectorPlacement.EquallySpacedRectSide\",\"uuid\":\"78580a51-84e7-4c5b-b2cf-22ca3fc7e95c\"}]},\"type\":\"ConnectorPlacement.EquallySpacedConnector\",\"uuid\":\"5e730262-b957-4973-b3fb-faaa2b08827c\"}],\"packageUris\":[\"http://schema.mathworks.com/mf0/Connector/R2020b\"],\"version\":\"1.0\"}"
  m_data_tdata : Outport
  m_data_tvalid : Outport  Port=2
  s_data_tready : Outport  Port=3
  wires:
  Relational/1 -> Mux/1
  s_data_tdata/1 -> Relational/2, Delay1/1
  Constant/1 -> Mux/3
  Mux/1 -> Mult/1, Mult/2
  Negate/1 -> m_data_tdata/1
  CMult/1 -> Mult1/2
  Constant1/1 -> Relational/1
  log2/1(m_data_tdata) -> CMult/1
  Mult/1 -> log2/1(s_data_tdata), Delay/1
  Delay1/1 -> Mux/2
  m_data_tready/1 -> s_data_tready/1, Logical/1
  s_data_tvalid/1 -> Logical1/2, Delay2/1, Logical/2
  Logical1/1 -> m_data_tvalid/1
  Logical/1 -> Delay1/2, Relational/3, Mux/4, Mult/3, log2/2(en), CMult/2, Mult1/3, Negate/2, Delay/2, Delay2/2
  Delay2/1 -> Logical1/1
  Delay/1 -> Mult1/1
  Mult1/1 -> Negate/1
